simulink library "Energy_converter_Electrical_to_Mechanical"  (R2016a)
settings: Solver=ode1  StartTime=0.0  StopTime=Inf  FixedStep=0.001  RelTol=1e-3
undefined symbols (not defined in the file): API1dcac_efficiency, API2dcac_efficiency, API3dcac_efficiency, aux_power_state, AWR_InvStError, dat, DiscIntNeverNeededParam, EDCU_p_RefTqeMOT, emot_AcCmprFront_inertia, emot_AcCmprFront_nTab_3rdD, emot_AcCmprFront_pwrAC, emot_AcCmprFront_Tau, emot_AcCmprFront_trqTab_2ndD, emot_AcCmprFront_vltTab_1stD, emot_AcCmprRear_inertia, emot_AcCmprRear_nTab_3rdD, emot_AcCmprRear_pwrAC, emot_AcCmprRear_Tau, emot_AcCmprRear_trqTab_2ndD, emot_AcCmprRear_vltTab_1stD, emot_AirCmpr_inertia, emot_AirCmpr_nTab_3rdD, emot_AirCmpr_pwrAC, emot_AirCmpr_Tau, emot_AirCmpr_trqTab_2ndD, emot_AirCmpr_vltTab_1stD, emot_aircomp_power, emot_Cth_rotor, emot_Cth_stator, emot_dtrqEmotNeg, emot_dtrqEmotPtv, emot_inv_pwracTab_1st, emot_inv_pwrDC, emot_inv_pwrLoss, emot_inv_VrmsTab_2nd, emot_j, emot_mot_pwrLoss, emot_nTab_1stD, emot_pwrEtaTab_nRow, emot_pwrEtaTab_pwrTab, emot_pwrEtaTab_trqClm, emot_Rth_rotor_oil, emot_Rth_stator_oil, emot_Rth_stator_rotor, emot_tractiongroup, emot_Trotor_init, emot_trqMaxRow, emot_trqMinRow, emot_Tstator_init, emot_vltTab_3rdD, FirstDrivenAxleNoOfEmot, inv_Cth_cooling_plate, inv_Cth_diode, inv_Cth_IGBT, inv_n_IGBT_per_Switch, inv_Rth_cooling_plate_coolant, inv_Rth_PS_cooling_plate, inv_Tplate_init, inv_Tpowerstack_init, midAxleNoOfEmot ... (+6)
libraries: Electrical_converter x12, Energy_converter_Electrical_to_Mechanical x12, simulink x7
(part 7 of 8)

== system Energy_converter_Electrical_to_Mechanical/AWR_DriveEmot_Gen2/AWR2_3/ZeroWhenNotReady2 ==
  Bus Creator4 : BusCreator  Inputs=11
  zero_EMD3_ACT_DcLinkVoltage : Constant  Value=0
  zero_EMD4_ACT_DcLinkPower : Constant  Value=0
  zero_EMD4_ACT_DigitalInput1 : Constant  Value=0
  zero_EMD4_ACT_InverterState : Constant  Value=0
  zero_EMD4_ACT_MaxJunctionTemperature : Constant  Value=0
  zero_EMD4_ACT_MaximumAvailableTorque : Constant  Value=0
  zero_EMD4_ACT_MotorSpeed : Constant  Value=0
  zero_EMD4_ACT_MotorTemperature : Constant  Value=0
  zero_EMD4_ACT_MotorTorque : Constant  Value=0
  zero_EMD4_ACT_ReferenceTorqueLimited : Constant  Value=0
  zero_trqEmot1DesPhy : Constant  Value=0
  Out1 : Outport
  wires:
  Bus Creator4/1 -> Out1/1  "awr3B"
  zero_EMD3_ACT_DcLinkVoltage/1 -> Bus Creator4/1  "EMD3_ACT_DcLinkVoltage"
  zero_EMD4_ACT_DigitalInput1/1 -> Bus Creator4/2  "EMD_ACT_DigitalInput1"
  zero_EMD4_ACT_MaximumAvailableTorque/1 -> Bus Creator4/3  "EMD_ACT_MaximumAvailableTorque"
  zero_EMD4_ACT_DcLinkPower/1 -> Bus Creator4/4  "EMD_ACT_DcLinkPower"
  zero_EMD4_ACT_MotorSpeed/1 -> Bus Creator4/5  "EMD_ACT_MotorSpeed"
  zero_EMD4_ACT_MotorTorque/1 -> Bus Creator4/6  "EMD_ACT_MotorTorque"
  zero_EMD4_ACT_InverterState/1 -> Bus Creator4/7  "EMD_ACT_InverterState"
  zero_EMD4_ACT_ReferenceTorqueLimited/1 -> Bus Creator4/8  "EMD_ACT_ReferenceTorqueLimited"
  zero_trqEmot1DesPhy/1 -> Bus Creator4/9  "trqEmotDesPhy"
  zero_EMD4_ACT_MaxJunctionTemperature/1 -> Bus Creator4/10  "EMD_ACT_MaxJunctionTemperature"
  zero_EMD4_ACT_MotorTemperature/1 -> Bus Creator4/11  "EMD_ACT_MotorTemperature"

== system Energy_converter_Electrical_to_Mechanical/AWR_DriveEmot_Gen2/EMD1_CMD_Command/Compare To Constant ==
  u : Inport
  Compare : RelationalOperator  Operator===  OutDataTypeStr=boolean  InputSameDT=on
  Constant : Constant  DisableCoverage=on  Value=const  OutDataTypeStr=Inherit: Inherit via back propagation
  y : Outport
  wires:
  Compare/1 -> y/1
  Constant/1 -> Compare/2
  u/1 -> Compare/1

== system Energy_converter_Electrical_to_Mechanical/AWR_DriveEmot_Gen2/EMD1_CMD_Command/Compare To Constant1 ==
  u : Inport
  Compare : RelationalOperator  Operator===  OutDataTypeStr=boolean  InputSameDT=on
  Constant : Constant  DisableCoverage=on  Value=const  OutDataTypeStr=Inherit: Inherit via back propagation
  y : Outport
  wires:
  Compare/1 -> y/1
  Constant/1 -> Compare/2
  u/1 -> Compare/1

== system Energy_converter_Electrical_to_Mechanical/AWR_DriveEmot_Gen2/EMD1_CMD_Command1/Compare To Constant ==
  u : Inport
  Compare : RelationalOperator  Operator===  OutDataTypeStr=boolean  InputSameDT=on
  Constant : Constant  DisableCoverage=on  Value=const  OutDataTypeStr=Inherit: Inherit via back propagation
  y : Outport
  wires:
  Compare/1 -> y/1
  Constant/1 -> Compare/2
  u/1 -> Compare/1

== system Energy_converter_Electrical_to_Mechanical/AWR_DriveEmot_Gen2/EMD1_CMD_Command1/Compare To Constant1 ==
  u : Inport
  Compare : RelationalOperator  Operator===  OutDataTypeStr=boolean  InputSameDT=on
  Constant : Constant  DisableCoverage=on  Value=const  OutDataTypeStr=Inherit: Inherit via back propagation
  y : Outport
  wires:
  Compare/1 -> y/1
  Constant/1 -> Compare/2
  u/1 -> Compare/1

== system Energy_converter_Electrical_to_Mechanical/AWR_DriveEmot_Gen2/EMD1_CMD_Command2/Compare To Constant ==
  u : Inport
  Compare : RelationalOperator  Operator===  OutDataTypeStr=boolean  InputSameDT=on
  Constant : Constant  DisableCoverage=on  Value=const  OutDataTypeStr=Inherit: Inherit via back propagation
  y : Outport
  wires:
  Compare/1 -> y/1
  Constant/1 -> Compare/2
  u/1 -> Compare/1

== system Energy_converter_Electrical_to_Mechanical/AWR_DriveEmot_Gen2/EMD1_CMD_Command2/Compare To Constant1 ==
  u : Inport
  Compare : RelationalOperator  Operator===  OutDataTypeStr=boolean  InputSameDT=on
  Constant : Constant  DisableCoverage=on  Value=const  OutDataTypeStr=Inherit: Inherit via back propagation
  y : Outport
  wires:
  Compare/1 -> y/1
  Constant/1 -> Compare/2
  u/1 -> Compare/1

== system Energy_converter_Electrical_to_Mechanical/AWR_DriveEmot_Gen2/EMD1_CMD_Command3/Compare To Constant ==
  u : Inport
  Compare : RelationalOperator  Operator===  OutDataTypeStr=boolean  InputSameDT=on
  Constant : Constant  DisableCoverage=on  Value=const  OutDataTypeStr=Inherit: Inherit via back propagation
  y : Outport
  wires:
  Compare/1 -> y/1
  Constant/1 -> Compare/2
  u/1 -> Compare/1

== system Energy_converter_Electrical_to_Mechanical/AWR_DriveEmot_Gen2/EMD1_CMD_Command3/Compare To Constant1 ==
  u : Inport
  Compare : RelationalOperator  Operator===  OutDataTypeStr=boolean  InputSameDT=on
  Constant : Constant  DisableCoverage=on  Value=const  OutDataTypeStr=Inherit: Inherit via back propagation
  y : Outport
  wires:
  Compare/1 -> y/1
  Constant/1 -> Compare/2
  u/1 -> Compare/1

== system Energy_converter_Electrical_to_Mechanical/AWR_DriveEmot_Gen2/SummarizeEmotorValuesForVehicle/Avoid_Div_by_zero ==
  U : Inport
  Constant : Constant  Value=10^-6
  Math Function : Math  Operator=reciprocal  SaturateOnIntegerOverflow=on
  Switch : Switch  Criteria=u2 > Threshold
  1/U : Outport
  wires:
  U/1 -> Math Function/1, Switch/2
  Constant/1 -> Switch/3
  Math Function/1 -> Switch/1
  Switch/1 -> 1/U/1

== system Energy_converter_Electrical_to_Mechanical/AWR_DriveEmot_edb_Data/AWR 1 TX/Nm_to_percent ==
  Nm_Torque : Inport
  Reference_Torque : Inport  Port=2
  Constant : Constant  Value=100
  Divide1 : Product  Inputs=*/
  Product1 : Product  RndMeth=Zero
  Torque_Percentage : Outport
  wires:
  Nm_Torque/1 -> Divide1/1  "Nm_Torque"
  Product1/1 -> Torque_Percentage/1  "Torque_Percentage"
  Reference_Torque/1 -> Divide1/2  "Reference_Torque"
  Divide1/1 -> Product1/1
  Constant/1 -> Product1/2

== system Energy_converter_Electrical_to_Mechanical/AWR_DriveEmot_edb_Data/AWR 1 TX/Nm_to_percent1 ==
  Nm_Torque : Inport
  Reference_Torque : Inport  Port=2
  Constant : Constant  Value=100
  Divide1 : Product  Inputs=*/
  Product1 : Product  RndMeth=Zero
  Torque_Percentage : Outport
  wires:
  Constant/1 -> Product1/2
  Divide1/1 -> Product1/1
  Reference_Torque/1 -> Divide1/2  "Reference_Torque"
  Product1/1 -> Torque_Percentage/1  "Torque_Percentage"
  Nm_Torque/1 -> Divide1/1  "Nm_Torque"

== system Energy_converter_Electrical_to_Mechanical/AWR_DriveEmot_edb_Data/AWR 1 TX/Nm_to_percent2 ==
  Nm_Torque : Inport
  Reference_Torque : Inport  Port=2
  Constant : Constant  Value=100
  Divide1 : Product  Inputs=*/
  Product1 : Product  RndMeth=Zero
  Torque_Percentage : Outport
  wires:
  Nm_Torque/1 -> Divide1/1  "Nm_Torque"
  Product1/1 -> Torque_Percentage/1  "Torque_Percentage"
  Reference_Torque/1 -> Divide1/2  "Reference_Torque"
  Divide1/1 -> Product1/1
  Constant/1 -> Product1/2

== system Energy_converter_Electrical_to_Mechanical/AWR_DriveEmot_edb_Data/AWR 2 TX/Nm_to_percent ==
  Nm_Torque : Inport
  Reference_Torque : Inport  Port=2
  Constant : Constant  Value=100
  Divide1 : Product  Inputs=*/
  Product1 : Product  RndMeth=Zero
  Torque_Percentage : Outport
  wires:
  Nm_Torque/1 -> Divide1/1  "Nm_Torque"
  Product1/1 -> Torque_Percentage/1  "Torque_Percentage"
  Reference_Torque/1 -> Divide1/2  "Reference_Torque"
  Divide1/1 -> Product1/1
  Constant/1 -> Product1/2

== system Energy_converter_Electrical_to_Mechanical/AWR_DriveEmot_edb_Data/AWR 2 TX/Nm_to_percent1 ==
  Nm_Torque : Inport
  Reference_Torque : Inport  Port=2
  Constant : Constant  Value=100
  Divide1 : Product  Inputs=*/
  Product1 : Product  RndMeth=Zero
  Torque_Percentage : Outport
  wires:
  Constant/1 -> Product1/2
  Divide1/1 -> Product1/1
  Reference_Torque/1 -> Divide1/2  "Reference_Torque"
  Product1/1 -> Torque_Percentage/1  "Torque_Percentage"
  Nm_Torque/1 -> Divide1/1  "Nm_Torque"

== system Energy_converter_Electrical_to_Mechanical/AWR_DriveEmot_edb_Data/AWR 2 TX/Nm_to_percent2 ==
  Nm_Torque : Inport
  Reference_Torque : Inport  Port=2
  Constant : Constant  Value=100
  Divide1 : Product  Inputs=*/
  Product1 : Product  RndMeth=Zero
  Torque_Percentage : Outport
  wires:
  Nm_Torque/1 -> Divide1/1  "Nm_Torque"
  Product1/1 -> Torque_Percentage/1  "Torque_Percentage"
  Reference_Torque/1 -> Divide1/2  "Reference_Torque"
  Divide1/1 -> Product1/1
  Constant/1 -> Product1/2

== system Energy_converter_Electrical_to_Mechanical/AWR_DriveEmot_edb_Data/AWR 3 TX/Nm_to_percent ==
  Nm_Torque : Inport
  Reference_Torque : Inport  Port=2
  Constant : Constant  Value=100
  Divide1 : Product  Inputs=*/
  Product1 : Product  RndMeth=Zero
  Torque_Percentage : Outport
  wires:
  Constant/1 -> Product1/2
  Divide1/1 -> Product1/1
  Reference_Torque/1 -> Divide1/2  "Reference_Torque"
  Product1/1 -> Torque_Percentage/1  "Torque_Percentage"
  Nm_Torque/1 -> Divide1/1  "Nm_Torque"

== system Energy_converter_Electrical_to_Mechanical/AWR_DriveEmot_edb_Data/AWR 3 TX/Nm_to_percent1 ==
  Nm_Torque : Inport
  Reference_Torque : Inport  Port=2
  Constant : Constant  Value=100
  Divide1 : Product  Inputs=*/
  Product1 : Product  RndMeth=Zero
  Torque_Percentage : Outport
  wires:
  Nm_Torque/1 -> Divide1/1  "Nm_Torque"
  Product1/1 -> Torque_Percentage/1  "Torque_Percentage"
  Reference_Torque/1 -> Divide1/2  "Reference_Torque"
  Divide1/1 -> Product1/1
  Constant/1 -> Product1/2

== system Energy_converter_Electrical_to_Mechanical/AWR_DriveEmot_edb_Data/AWR 3 TX/Nm_to_percent2 ==
  Nm_Torque : Inport
  Reference_Torque : Inport  Port=2
  Constant : Constant  Value=100
  Divide1 : Product  Inputs=*/
  Product1 : Product  RndMeth=Zero
  Torque_Percentage : Outport
  wires:
  Constant/1 -> Product1/2
  Divide1/1 -> Product1/1
  Reference_Torque/1 -> Divide1/2  "Reference_Torque"
  Product1/1 -> Torque_Percentage/1  "Torque_Percentage"
  Nm_Torque/1 -> Divide1/1  "Nm_Torque"

== system Energy_converter_Electrical_to_Mechanical/AWR_DriveEmot_edb_Data/AWR 4 TX/Nm_to_percent ==
  Nm_Torque : Inport
  Reference_Torque : Inport  Port=2
  Constant : Constant  Value=100
  Divide1 : Product  Inputs=*/
  Product1 : Product  RndMeth=Zero
  Torque_Percentage : Outport
  wires:
  Nm_Torque/1 -> Divide1/1  "Nm_Torque"
  Product1/1 -> Torque_Percentage/1  "Torque_Percentage"
  Reference_Torque/1 -> Divide1/2  "Reference_Torque"
  Divide1/1 -> Product1/1
  Constant/1 -> Product1/2

== system Energy_converter_Electrical_to_Mechanical/AWR_DriveEmot_edb_Data/AWR 4 TX/Nm_to_percent1 ==
  Nm_Torque : Inport
  Reference_Torque : Inport  Port=2
  Constant : Constant  Value=100
  Divide1 : Product  Inputs=*/
  Product1 : Product  RndMeth=Zero
  Torque_Percentage : Outport
  wires:
  Constant/1 -> Product1/2
  Divide1/1 -> Product1/1
  Reference_Torque/1 -> Divide1/2  "Reference_Torque"
  Product1/1 -> Torque_Percentage/1  "Torque_Percentage"
  Nm_Torque/1 -> Divide1/1  "Nm_Torque"

== system Energy_converter_Electrical_to_Mechanical/AWR_DriveEmot_edb_Data/AWR 4 TX/Nm_to_percent2 ==
  Nm_Torque : Inport
  Reference_Torque : Inport  Port=2
  Constant : Constant  Value=100
  Divide1 : Product  Inputs=*/
  Product1 : Product  RndMeth=Zero
  Torque_Percentage : Outport
  wires:
  Nm_Torque/1 -> Divide1/1  "Nm_Torque"
  Product1/1 -> Torque_Percentage/1  "Torque_Percentage"
  Reference_Torque/1 -> Divide1/2  "Reference_Torque"
  Divide1/1 -> Product1/1
  Constant/1 -> Product1/2

== system Energy_converter_Electrical_to_Mechanical/AWR_DriveEmot_edb_Data/AWR1_4/ZeroWhenNotReady1 ==
  Bus Creator4 : BusCreator  Inputs=11
  zero_EMD1_ACT_DcLinkPower : Constant  Value=0
  zero_EMD1_ACT_DcLinkVoltage : Constant  Value=0
  zero_EMD1_ACT_DigitalInput1 : Constant  Value=0
  zero_EMD1_ACT_InverterState : Constant  Value=0
  zero_EMD1_ACT_MaxJunctionTemperature : Constant  Value=0
  zero_EMD1_ACT_MaximumAvailableTorque : Constant  Value=0
  zero_EMD1_ACT_MotorSpeed : Constant  Value=0
  zero_EMD1_ACT_MotorTemperature : Constant  Value=0
  zero_EMD1_ACT_MotorTorque : Constant  Value=0
  zero_EMD1_ACT_ReferenceTorqueLimited : Constant  Value=0
  zero_trqEmot1DesPhy : Constant  Value=0
  Out1 : Outport
  wires:
  Bus Creator4/1 -> Out1/1  "awr1B"
  zero_EMD1_ACT_DcLinkVoltage/1 -> Bus Creator4/1  "EMD1_ACT_DcLinkVoltage"
  zero_EMD1_ACT_DigitalInput1/1 -> Bus Creator4/2  "EMD_ACT_DigitalInput1"
  zero_EMD1_ACT_MaximumAvailableTorque/1 -> Bus Creator4/3  "EMD_ACT_MaximumAvailableTorque"
  zero_EMD1_ACT_DcLinkPower/1 -> Bus Creator4/4  "EMD_ACT_DcLinkPower"
  zero_EMD1_ACT_MotorSpeed/1 -> Bus Creator4/5  "EMD_ACT_MotorSpeed"
  zero_EMD1_ACT_MotorTorque/1 -> Bus Creator4/6  "EMD_ACT_MotorTorque"
  zero_EMD1_ACT_InverterState/1 -> Bus Creator4/7  "EMD_ACT_InverterState"
  zero_EMD1_ACT_ReferenceTorqueLimited/1 -> Bus Creator4/8  "EMD_ACT_ReferenceTorqueLimited"
  zero_trqEmot1DesPhy/1 -> Bus Creator4/9  "trqEmotDesPhy"
  zero_EMD1_ACT_MaxJunctionTemperature/1 -> Bus Creator4/10  "EMD_ACT_MaxJunctionTemperature"
  zero_EMD1_ACT_MotorTemperature/1 -> Bus Creator4/11  "EMD_ACT_MotorTemperature"

== system Energy_converter_Electrical_to_Mechanical/AWR_DriveEmot_edb_Data/AWR1_4/ZeroWhenNotReady2 ==
  Bus Creator4 : BusCreator  Inputs=11
  zero_EMD4_ACT_DcLinkPower : Constant  Value=0
  zero_EMD4_ACT_DcLinkVoltage : Constant  Value=0
  zero_EMD4_ACT_DigitalInput1 : Constant  Value=0
  zero_EMD4_ACT_InverterState : Constant  Value=0
  zero_EMD4_ACT_MaxJunctionTemperature : Constant  Value=0
  zero_EMD4_ACT_MaximumAvailableTorque : Constant  Value=0
  zero_EMD4_ACT_MotorSpeed : Constant  Value=0
  zero_EMD4_ACT_MotorTemperature : Constant  Value=0
  zero_EMD4_ACT_MotorTorque : Constant  Value=0
  zero_EMD4_ACT_ReferenceTorqueLimited : Constant  Value=0
  zero_trqEmot1DesPhy : Constant  Value=0
  Out1 : Outport
  wires:
  zero_EMD4_ACT_MotorTemperature/1 -> Bus Creator4/11  "EMD_ACT_MotorTemperature"
  zero_EMD4_ACT_MaxJunctionTemperature/1 -> Bus Creator4/10  "EMD_ACT_MaxJunctionTemperature"
  zero_trqEmot1DesPhy/1 -> Bus Creator4/9  "trqEmotDesPhy"
  zero_EMD4_ACT_ReferenceTorqueLimited/1 -> Bus Creator4/8  "EMD_ACT_ReferenceTorqueLimited"
  zero_EMD4_ACT_InverterState/1 -> Bus Creator4/7  "EMD_ACT_InverterState"
  zero_EMD4_ACT_MotorTorque/1 -> Bus Creator4/6  "EMD_ACT_MotorTorque"
  zero_EMD4_ACT_MotorSpeed/1 -> Bus Creator4/5  "EMD_ACT_MotorSpeed"
  zero_EMD4_ACT_DcLinkPower/1 -> Bus Creator4/4  "EMD_ACT_DcLinkPower"
  zero_EMD4_ACT_MaximumAvailableTorque/1 -> Bus Creator4/3  "EMD_ACT_MaximumAvailableTorque"
  zero_EMD4_ACT_DigitalInput1/1 -> Bus Creator4/2  "EMD_ACT_DigitalInput1"
  zero_EMD4_ACT_DcLinkVoltage/1 -> Bus Creator4/1  "EMD4_ACT_DcLinkVoltage"
  Bus Creator4/1 -> Out1/1  "awr1B"

== system Energy_converter_Electrical_to_Mechanical/AWR_DriveEmot_edb_Data/AWR2_3/ZeroWhenNotReady1 ==
  Bus Creator4 : BusCreator  Inputs=11
  zero_EMD1_ACT_DcLinkPower : Constant  Value=0
  zero_EMD1_ACT_DigitalInput1 : Constant  Value=0
  zero_EMD1_ACT_InverterState : Constant  Value=0
  zero_EMD1_ACT_MaxJunctionTemperature : Constant  Value=0
  zero_EMD1_ACT_MaximumAvailableTorque : Constant  Value=0
  zero_EMD1_ACT_MotorSpeed : Constant  Value=0
  zero_EMD1_ACT_MotorTemperature : Constant  Value=0
  zero_EMD1_ACT_MotorTorque : Constant  Value=0
  zero_EMD1_ACT_ReferenceTorqueLimited : Constant  Value=0
  zero_EMD2_ACT_DcLinkVoltage : Constant  Value=0
  zero_trqEmot1DesPhy : Constant  Value=0
  Out1 : Outport
  wires:
  zero_EMD1_ACT_MotorTemperature/1 -> Bus Creator4/11  "EMD_ACT_MotorTemperature"
  zero_EMD1_ACT_MaxJunctionTemperature/1 -> Bus Creator4/10  "EMD_ACT_MaxJunctionTemperature"
  zero_trqEmot1DesPhy/1 -> Bus Creator4/9  "trqEmotDesPhy"
  zero_EMD1_ACT_ReferenceTorqueLimited/1 -> Bus Creator4/8  "EMD_ACT_ReferenceTorqueLimited"
  zero_EMD1_ACT_InverterState/1 -> Bus Creator4/7  "EMD_ACT_InverterState"
  zero_EMD1_ACT_MotorTorque/1 -> Bus Creator4/6  "EMD_ACT_MotorTorque"
  zero_EMD1_ACT_MotorSpeed/1 -> Bus Creator4/5  "EMD_ACT_MotorSpeed"
  zero_EMD1_ACT_DcLinkPower/1 -> Bus Creator4/4  "EMD_ACT_DcLinkPower"
  zero_EMD1_ACT_MaximumAvailableTorque/1 -> Bus Creator4/3  "EMD_ACT_MaximumAvailableTorque"
  zero_EMD1_ACT_DigitalInput1/1 -> Bus Creator4/2  "EMD_ACT_DigitalInput1"
  zero_EMD2_ACT_DcLinkVoltage/1 -> Bus Creator4/1  "EMD2_ACT_DcLinkVoltage"
  Bus Creator4/1 -> Out1/1  "awr2B"

== system Energy_converter_Electrical_to_Mechanical/AWR_DriveEmot_edb_Data/AWR2_3/ZeroWhenNotReady2 ==
  Bus Creator4 : BusCreator  Inputs=11
  zero_EMD3_ACT_DcLinkVoltage : Constant  Value=0
  zero_EMD4_ACT_DcLinkPower : Constant  Value=0
  zero_EMD4_ACT_DigitalInput1 : Constant  Value=0
  zero_EMD4_ACT_InverterState : Constant  Value=0
  zero_EMD4_ACT_MaxJunctionTemperature : Constant  Value=0
  zero_EMD4_ACT_MaximumAvailableTorque : Constant  Value=0
  zero_EMD4_ACT_MotorSpeed : Constant  Value=0
  zero_EMD4_ACT_MotorTemperature : Constant  Value=0
  zero_EMD4_ACT_MotorTorque : Constant  Value=0
  zero_EMD4_ACT_ReferenceTorqueLimited : Constant  Value=0
  zero_trqEmot1DesPhy : Constant  Value=0
  Out1 : Outport
  wires:
  Bus Creator4/1 -> Out1/1  "awr3B"
  zero_EMD3_ACT_DcLinkVoltage/1 -> Bus Creator4/1  "EMD3_ACT_DcLinkVoltage"
  zero_EMD4_ACT_DigitalInput1/1 -> Bus Creator4/2  "EMD_ACT_DigitalInput1"
  zero_EMD4_ACT_MaximumAvailableTorque/1 -> Bus Creator4/3  "EMD_ACT_MaximumAvailableTorque"
  zero_EMD4_ACT_DcLinkPower/1 -> Bus Creator4/4  "EMD_ACT_DcLinkPower"
  zero_EMD4_ACT_MotorSpeed/1 -> Bus Creator4/5  "EMD_ACT_MotorSpeed"
  zero_EMD4_ACT_MotorTorque/1 -> Bus Creator4/6  "EMD_ACT_MotorTorque"
  zero_EMD4_ACT_InverterState/1 -> Bus Creator4/7  "EMD_ACT_InverterState"
  zero_EMD4_ACT_ReferenceTorqueLimited/1 -> Bus Creator4/8  "EMD_ACT_ReferenceTorqueLimited"
  zero_trqEmot1DesPhy/1 -> Bus Creator4/9  "trqEmotDesPhy"
  zero_EMD4_ACT_MaxJunctionTemperature/1 -> Bus Creator4/10  "EMD_ACT_MaxJunctionTemperature"
  zero_EMD4_ACT_MotorTemperature/1 -> Bus Creator4/11  "EMD_ACT_MotorTemperature"

== system Energy_converter_Electrical_to_Mechanical/AWR_DriveEmot_edb_Data/EMD1_CMD_Command/Compare To Constant ==
  u : Inport
  Compare : RelationalOperator  Operator===  OutDataTypeStr=boolean  InputSameDT=on
  Constant : Constant  DisableCoverage=on  Value=const  OutDataTypeStr=Inherit: Inherit via back propagation
  y : Outport
  wires:
  Compare/1 -> y/1
  Constant/1 -> Compare/2
  u/1 -> Compare/1

== system Energy_converter_Electrical_to_Mechanical/AWR_DriveEmot_edb_Data/EMD1_CMD_Command/Compare To Constant1 ==
  u : Inport
  Compare : RelationalOperator  Operator===  OutDataTypeStr=boolean  InputSameDT=on
  Constant : Constant  DisableCoverage=on  Value=const  OutDataTypeStr=Inherit: Inherit via back propagation
  y : Outport
  wires:
  Compare/1 -> y/1
  Constant/1 -> Compare/2
  u/1 -> Compare/1

== system Energy_converter_Electrical_to_Mechanical/AWR_DriveEmot_edb_Data/EMD1_CMD_Command1/Compare To Constant ==
  u : Inport
  Compare : RelationalOperator  Operator===  OutDataTypeStr=boolean  InputSameDT=on
  Constant : Constant  DisableCoverage=on  Value=const  OutDataTypeStr=Inherit: Inherit via back propagation
  y : Outport
  wires:
  Compare/1 -> y/1
  Constant/1 -> Compare/2
  u/1 -> Compare/1

== system Energy_converter_Electrical_to_Mechanical/AWR_DriveEmot_edb_Data/EMD1_CMD_Command1/Compare To Constant1 ==
  u : Inport
  Compare : RelationalOperator  Operator===  OutDataTypeStr=boolean  InputSameDT=on
  Constant : Constant  DisableCoverage=on  Value=const  OutDataTypeStr=Inherit: Inherit via back propagation
  y : Outport
  wires:
  Compare/1 -> y/1
  Constant/1 -> Compare/2
  u/1 -> Compare/1

== system Energy_converter_Electrical_to_Mechanical/AWR_DriveEmot_edb_Data/EMD1_CMD_Command2/Compare To Constant ==
  u : Inport
  Compare : RelationalOperator  Operator===  OutDataTypeStr=boolean  InputSameDT=on
  Constant : Constant  DisableCoverage=on  Value=const  OutDataTypeStr=Inherit: Inherit via back propagation
  y : Outport
  wires:
  Compare/1 -> y/1
  Constant/1 -> Compare/2
  u/1 -> Compare/1

== system Energy_converter_Electrical_to_Mechanical/AWR_DriveEmot_edb_Data/EMD1_CMD_Command2/Compare To Constant1 ==
  u : Inport
  Compare : RelationalOperator  Operator===  OutDataTypeStr=boolean  InputSameDT=on
  Constant : Constant  DisableCoverage=on  Value=const  OutDataTypeStr=Inherit: Inherit via back propagation
  y : Outport
  wires:
  Compare/1 -> y/1
  Constant/1 -> Compare/2
  u/1 -> Compare/1

== system Energy_converter_Electrical_to_Mechanical/AWR_DriveEmot_edb_Data/EMD1_CMD_Command3/Compare To Constant ==
  u : Inport
  Compare : RelationalOperator  Operator===  OutDataTypeStr=boolean  InputSameDT=on
  Constant : Constant  DisableCoverage=on  Value=const  OutDataTypeStr=Inherit: Inherit via back propagation
  y : Outport
  wires:
  Compare/1 -> y/1
  Constant/1 -> Compare/2
  u/1 -> Compare/1

== system Energy_converter_Electrical_to_Mechanical/AWR_DriveEmot_edb_Data/EMD1_CMD_Command3/Compare To Constant1 ==
  u : Inport
  Compare : RelationalOperator  Operator===  OutDataTypeStr=boolean  InputSameDT=on
  Constant : Constant  DisableCoverage=on  Value=const  OutDataTypeStr=Inherit: Inherit via back propagation
  y : Outport
  wires:
  Compare/1 -> y/1
  Constant/1 -> Compare/2
  u/1 -> Compare/1

== system Energy_converter_Electrical_to_Mechanical/AWR_DriveEmot_edb_Data/SummarizeEmotorValuesForVehicle/Avoid_Div_by_zero ==
  U : Inport
  Constant : Constant  Value=10^-6
  Math Function : Math  Operator=reciprocal  SaturateOnIntegerOverflow=on
  Switch : Switch  Criteria=u2 > Threshold
  1/U : Outport
  wires:
  U/1 -> Math Function/1, Switch/2
  Constant/1 -> Switch/3
  Math Function/1 -> Switch/1
  Switch/1 -> 1/U/1

== system Energy_converter_Electrical_to_Mechanical/GTR_Electric_machine/Thermal/Cooling2 ==
  power loss : Inport
  cooling inlet : Inport  Port=2
  Add1 : Sum  Inputs=-+
  Add2 : Sum  Inputs=-+
  Bus Selector : BusSelector  OutputSignals=mass flow [kg/s],temperature [K]
  Gain : Gain  Gain=1/dat.Rth.value
  Gain1 : Gain  Gain=1/dat.cm.value
  Integrator : Integrator  InitialCondition=hilsmdl.init.temp.value
  Mux : Mux  Inputs=3
  Mux1 : Mux  Inputs=2
  calc mean temperature : Fcn  Expr=dat.alpha.value*u(1) + (1-dat.alpha.value)*u(2)
  calc outlet temperature : Fcn  Expr=(u(3)+u(2)*(dat.Rth.value*dat.coolingFluid.c.value*u(1)-dat.alpha.value)) / (1+dat.Rth.value*dat.coolingFluid.c.value*u(1)-dat.alpha.value)
  internal temperature : Outport
  fluid outlet temperature : Outport  Port=2
  wires:
  Mux/1 -> calc outlet temperature/1
  calc outlet temperature/1 -> Mux1/2, fluid outlet temperature/1  "fluid outlet temperature [K]"
  Bus Selector/2 -> Mux1/1, Mux/2  "<temperature [K]>"
  Add1/1 -> Gain/1
  Gain/1 -> Add2/1  "P cooling [W]"
  Add2/1 -> Gain1/1
  Gain1/1 -> Integrator/1
  Integrator/1 -> Mux/3, Add1/2, internal temperature/1  "internal temperature [K]"
  cooling inlet/1 -> Bus Selector/1
  power loss/1 -> Add2/2  "power loss [W]"
  Mux1/1 -> calc mean temperature/1
  calc mean temperature/1 -> Add1/1  "T_mean [K]"
  Bus Selector/1 -> Mux/1  "<mass flow [kg/s]>"

== system Energy_converter_Electrical_to_Mechanical/GTR_Electric_machine/local controller/PI controller ==
  RefSpeed : Inport
  ActSpeed : Inport  Port=2
  Reset : Inport  Port=3
  Gain : Gain  Gain=dat.controller.i.value
  Gain2 : Gain  Gain=dat.controller.p.value
  Integrator : Integrator  ExternalReset=either
  Product : Product  RndMeth=Zero
  Sum : Sum  Inputs=|+-
  Sum1 : Sum  Inputs=|++
  Ctrl signal : Outport
  wires:
  Sum1/1 -> Ctrl signal/1
  Reset/1 -> Integrator/2, Product/2
  ActSpeed/1 -> Sum/2
  RefSpeed/1 -> Sum/1
  Product/1 -> Integrator/1
  Gain/1 -> Product/1
  Gain2/1 -> Sum1/2
  Integrator/1 -> Sum1/1
  Sum/1 -> Gain2/1, Gain/1

== system Energy_converter_Electrical_to_Mechanical/e-Motor/Thermic_Model_Inverter/C_IGBT_and_Diode ==
  P_Heat_eff : Inport
  T : Inport  Port=2
  Add : Sum
  Clock : Clock
  Divide : Product  Inputs=*/
  Heat_Capacity_PowerStack [J/K] : Constant  Value=inv_Cth_IGBT+inv_Cth_diode
  Product : Product
  Product1 : Product
  Sum : Sum  Inputs=|+-
  Unit Delay : UnitDelay  SampleTime=-1
  T_new : Outport
  wires:
  Sum/1 -> Product/2  "[s]"
  P_Heat_eff/1 -> Product/1
  Product/1 -> Add/1  "[J]"
  T/1 -> Product1/1  "[K]"
  Heat_Capacity_PowerStack [J/K]/1 -> Product1/2, Divide/2
  Product1/1 -> Add/2  "[J]"
  Add/1 -> Divide/1
  Divide/1 -> T_new/1  "[K]"
  Clock/1 -> Sum/1, Unit Delay/1
  Unit Delay/1 -> Sum/2

== system Energy_converter_Electrical_to_Mechanical/e-Motor/Thermic_Model_Inverter/C_Plate ==
  P_Heat_eff : Inport
  T : Inport  Port=2
  Add : Sum
  Clock : Clock
  Divide : Product  Inputs=*/
  Heat_Capacity_Plate [J/K] : Constant  Value=inv_Cth_cooling_plate
  Product : Product
  Product1 : Product
  Sum : Sum  Inputs=|+-
  Unit Delay : UnitDelay  SampleTime=-1
  T_new : Outport
  wires:
  Sum/1 -> Product/2  "[s]"
  P_Heat_eff/1 -> Product/1
  Product/1 -> Add/1  "[J]"
  T/1 -> Product1/1  "[K]"
  Product1/1 -> Add/2  "[J]"
  Add/1 -> Divide/1
  Divide/1 -> T_new/1  "[K]"
  Heat_Capacity_Plate [J/K]/1 -> Product1/2, Divide/2
  Clock/1 -> Sum/1, Unit Delay/1
  Unit Delay/1 -> Sum/2

== system Energy_converter_Electrical_to_Mechanical/e-Motor/Thermic_Model_Inverter/R_PS-Plate ==
  T_IGBT : Inport
  T_Plate : Inport  Port=2
  Add : Sum  Inputs=+-
  Divide : Product  Inputs=*/
  R_th_IGBT_Plate : Constant  Value=inv_Rth_PS_cooling_plate
  dQ : Outport
  wires:
  R_th_IGBT_Plate/1 -> Divide/2
  Divide/1 -> dQ/1
  Add/1 -> Divide/1
  T_Plate/1 -> Add/2
  T_IGBT/1 -> Add/1

== system Energy_converter_Electrical_to_Mechanical/e-Motor/Thermic_Model_Inverter/R_Plate-Coolant ==
  T_Plate : Inport
  T_Coolant : Inport  Port=2
  Add : Sum  Inputs=+-
  Divide : Product  Inputs=*/
  Rth_cooling_plate_coolant : Constant  Value=inv_Rth_cooling_plate_coolant
  dQ : Outport
  wires:
  T_Plate/1 -> Add/1
  T_Coolant/1 -> Add/2
  Add/1 -> Divide/1
  Divide/1 -> dQ/1
  Rth_cooling_plate_coolant/1 -> Divide/2

== system Energy_converter_Electrical_to_Mechanical/e-Motor/Thermic_Model_PMSM_slot2/C_Rotor ==
  P_Heat_eff : Inport
  T : Inport  Port=2
  Add : Sum
  Clock : Clock
  Divide : Product  Inputs=*/
  Heat_Capacity_Rotor [J/K] : Constant  Value=emot_Cth_rotor
  Product : Product
  Product1 : Product
  Sum : Sum  Inputs=|+-
  Unit Delay : UnitDelay  SampleTime=-1
  T_new : Outport
  wires:
  Divide/1 -> T_new/1  "[K]"
  Add/1 -> Divide/1
  Product1/1 -> Add/2  "[J]"
  Heat_Capacity_Rotor [J/K]/1 -> Divide/2, Product1/2
  T/1 -> Product1/1  "[K]"
  Product/1 -> Add/1  "[J]"
  P_Heat_eff/1 -> Product/1
  Sum/1 -> Product/2  "[s]"
  Clock/1 -> Sum/1, Unit Delay/1
  Unit Delay/1 -> Sum/2

== system Energy_converter_Electrical_to_Mechanical/e-Motor/Thermic_Model_PMSM_slot2/C_Stator ==
  P_Heat_eff : Inport
  T : Inport  Port=2
  Add : Sum
  Clock : Clock
  Divide : Product  Inputs=*/
  Heat_Capacity_Stator [J/K] : Constant  Value=emot_Cth_stator
  Product : Product
  Product1 : Product
  Sum : Sum  Inputs=|+-
  Unit Delay : UnitDelay  SampleTime=-1
  T_new : Outport
  wires:
  Sum/1 -> Product/2  "[s]"
  P_Heat_eff/1 -> Product/1
  Product/1 -> Add/1  "[J]"
  T/1 -> Product1/1  "[K]"
  Heat_Capacity_Stator [J/K]/1 -> Product1/2, Divide/2
  Product1/1 -> Add/2  "[J]"
  Add/1 -> Divide/1
  Divide/1 -> T_new/1  "[K]"
  Clock/1 -> Sum/1, Unit Delay/1
  Unit Delay/1 -> Sum/2

== system Energy_converter_Electrical_to_Mechanical/e-Motor/Thermic_Model_PMSM_slot2/K2degC ==
  In1 : Inport
  Add : Sum  Inputs=+-
  Constant : Constant  Value=273.15
  Out1 : Outport
  wires:
  In1/1 -> Add/1
  Add/1 -> Out1/1
  Constant/1 -> Add/2

== system Energy_converter_Electrical_to_Mechanical/e-Motor/Thermic_Model_PMSM_slot2/K2degC1 ==
  In1 : Inport
  Add : Sum  Inputs=+-
  Constant : Constant  Value=273.15
  Out1 : Outport
  wires:
  In1/1 -> Add/1
  Add/1 -> Out1/1
  Constant/1 -> Add/2

== system Energy_converter_Electrical_to_Mechanical/e-Motor/Thermic_Model_PMSM_slot2/R_RotorOil ==
  T_Rotor : Inport
  T_Oil : Inport  Port=2
  Add : Sum  Inputs=+-
  Divide : Product  Inputs=*/
  R_th_Rot_Oil : Constant  Value=emot_Rth_rotor_oil
  dQ : Outport
  wires:
  T_Rotor/1 -> Add/1
  T_Oil/1 -> Add/2
  Add/1 -> Divide/1
  Divide/1 -> dQ/1
  R_th_Rot_Oil/1 -> Divide/2

== system Energy_converter_Electrical_to_Mechanical/e-Motor/Thermic_Model_PMSM_slot2/R_StatorOil ==
  T_Oil : Inport
  T_Stator : Inport  Port=2
  Add : Sum  Inputs=-+
  Divide : Product  Inputs=*/
  R_th_Stat_Oil : Constant  Value=emot_Rth_stator_oil
  dQ : Outport
  wires:
  T_Oil/1 -> Add/1
  T_Stator/1 -> Add/2
  Add/1 -> Divide/1
  Divide/1 -> dQ/1
  R_th_Stat_Oil/1 -> Divide/2

== system Energy_converter_Electrical_to_Mechanical/e-Motor/Thermic_Model_PMSM_slot2/R_StatorRotor ==
  T_Stator : Inport
  T_Rotor : Inport  Port=2
  Add : Sum  Inputs=+-
  Divide : Product  Inputs=*/
  R_th_Stat_Rot : Constant  Value=emot_Rth_stator_rotor
  dQ : Outport
  wires:
  R_th_Stat_Rot/1 -> Divide/2
  Divide/1 -> dQ/1
  Add/1 -> Divide/1
  T_Rotor/1 -> Add/2
  T_Stator/1 -> Add/1

== system Energy_converter_Electrical_to_Mechanical/e-Motor/Thermic_Model_PMSM_slot2/degC2K ==
  In1 : Inport
  Add : Sum
  Constant : Constant  Value=273.15
  Out1 : Outport
  wires:
  In1/1 -> Add/1
  Add/1 -> Out1/1
  Constant/1 -> Add/2

== system Energy_converter_Electrical_to_Mechanical/e-Motor/Thermic_Model_PMSM_slot2/degC2K1 ==
  In1 : Inport
  Add : Sum
  Constant : Constant  Value=273.15
  Out1 : Outport
  wires:
  Constant/1 -> Add/2
  Add/1 -> Out1/1
  In1/1 -> Add/1

== system Energy_converter_Electrical_to_Mechanical/e-Motor/Thermic_Model_PMSM_slot2/degC2K2 ==
  In1 : Inport
  Add : Sum
  Constant : Constant  Value=273.15
  Out1 : Outport
  wires:
  In1/1 -> Add/1
  Add/1 -> Out1/1
  Constant/1 -> Add/2

== system Energy_converter_Electrical_to_Mechanical/e-Motor_Gen2/Thermic_Model_Inverter/C_IGBT_and_Diode ==
  P_Heat_eff : Inport
  T : Inport  Port=2
  Add : Sum
  Clock : Clock
  Divide : Product  Inputs=*/
  Heat_Capacity_PowerStack [J/K] : Constant  Value=inv_Cth_IGBT+inv_Cth_diode
  Product : Product
  Product1 : Product
  Sum : Sum  Inputs=|+-
  Unit Delay : UnitDelay  SampleTime=-1
  T_new : Outport
  wires:
  Sum/1 -> Product/2  "[s]"
  P_Heat_eff/1 -> Product/1
  Product/1 -> Add/1  "[J]"
  T/1 -> Product1/1  "[K]"
  Heat_Capacity_PowerStack [J/K]/1 -> Product1/2, Divide/2
  Product1/1 -> Add/2  "[J]"
  Add/1 -> Divide/1
  Divide/1 -> T_new/1  "[K]"
  Clock/1 -> Sum/1, Unit Delay/1
  Unit Delay/1 -> Sum/2

== system Energy_converter_Electrical_to_Mechanical/e-Motor_Gen2/Thermic_Model_Inverter/C_Plate ==
  P_Heat_eff : Inport
  T : Inport  Port=2
  Add : Sum
  Clock : Clock
  Divide : Product  Inputs=*/
  Heat_Capacity_Plate [J/K] : Constant  Value=inv_Cth_cooling_plate
  Product : Product
  Product1 : Product
  Sum : Sum  Inputs=|+-
  Unit Delay : UnitDelay  SampleTime=-1
  T_new : Outport
  wires:
  Sum/1 -> Product/2  "[s]"
  P_Heat_eff/1 -> Product/1
  Product/1 -> Add/1  "[J]"
  T/1 -> Product1/1  "[K]"
  Product1/1 -> Add/2  "[J]"
  Add/1 -> Divide/1
  Divide/1 -> T_new/1  "[K]"
  Heat_Capacity_Plate [J/K]/1 -> Product1/2, Divide/2
  Clock/1 -> Sum/1, Unit Delay/1
  Unit Delay/1 -> Sum/2

== system Energy_converter_Electrical_to_Mechanical/e-Motor_Gen2/Thermic_Model_Inverter/R_PS-Plate ==
  T_IGBT : Inport
  T_Plate : Inport  Port=2
  Add : Sum  Inputs=+-
  Divide : Product  Inputs=*/
  R_th_IGBT_Plate : Constant  Value=inv_Rth_PS_cooling_plate
  dQ : Outport
  wires:
  R_th_IGBT_Plate/1 -> Divide/2
  Divide/1 -> dQ/1
  Add/1 -> Divide/1
  T_Plate/1 -> Add/2
  T_IGBT/1 -> Add/1

== system Energy_converter_Electrical_to_Mechanical/e-Motor_Gen2/Thermic_Model_Inverter/R_Plate-Coolant ==
  T_Plate : Inport
  T_Coolant : Inport  Port=2
  Add : Sum  Inputs=+-
  Divide : Product  Inputs=*/
  Rth_cooling_plate_coolant : Constant  Value=inv_Rth_cooling_plate_coolant
  dQ : Outport
  wires:
  T_Plate/1 -> Add/1
  T_Coolant/1 -> Add/2
  Add/1 -> Divide/1
  Divide/1 -> dQ/1
  Rth_cooling_plate_coolant/1 -> Divide/2

== system Energy_converter_Electrical_to_Mechanical/e-Motor_Gen2/Thermic_Model_PMSM_slot2/C_Rotor ==
  P_Heat_eff : Inport
  T : Inport  Port=2
  Add : Sum
  Clock : Clock
  Divide : Product  Inputs=*/
  Heat_Capacity_Rotor [J/K] : Constant  Value=emot_Cth_rotor
  Product : Product
  Product1 : Product
  Sum : Sum  Inputs=|+-
  Unit Delay : UnitDelay  SampleTime=-1
  T_new : Outport
  wires:
  Divide/1 -> T_new/1  "[K]"
  Add/1 -> Divide/1
  Product1/1 -> Add/2  "[J]"
  Heat_Capacity_Rotor [J/K]/1 -> Divide/2, Product1/2
  T/1 -> Product1/1  "[K]"
  Product/1 -> Add/1  "[J]"
  P_Heat_eff/1 -> Product/1
  Sum/1 -> Product/2  "[s]"
  Clock/1 -> Sum/1, Unit Delay/1
  Unit Delay/1 -> Sum/2

== system Energy_converter_Electrical_to_Mechanical/e-Motor_Gen2/Thermic_Model_PMSM_slot2/C_Stator ==
  P_Heat_eff : Inport
  T : Inport  Port=2
  Add : Sum
  Clock : Clock
  Divide : Product  Inputs=*/
  Heat_Capacity_Stator [J/K] : Constant  Value=emot_Cth_stator
  Product : Product
  Product1 : Product
  Sum : Sum  Inputs=|+-
  Unit Delay : UnitDelay  SampleTime=-1
  T_new : Outport
  wires:
  Sum/1 -> Product/2  "[s]"
  P_Heat_eff/1 -> Product/1
  Product/1 -> Add/1  "[J]"
  T/1 -> Product1/1  "[K]"
  Heat_Capacity_Stator [J/K]/1 -> Product1/2, Divide/2
  Product1/1 -> Add/2  "[J]"
  Add/1 -> Divide/1
  Divide/1 -> T_new/1  "[K]"
  Clock/1 -> Sum/1, Unit Delay/1
  Unit Delay/1 -> Sum/2

== system Energy_converter_Electrical_to_Mechanical/e-Motor_Gen2/Thermic_Model_PMSM_slot2/K2degC ==
  In1 : Inport
  Add : Sum  Inputs=+-
  Constant : Constant  Value=273.15
  Out1 : Outport
  wires:
  In1/1 -> Add/1
  Add/1 -> Out1/1
  Constant/1 -> Add/2

== system Energy_converter_Electrical_to_Mechanical/e-Motor_Gen2/Thermic_Model_PMSM_slot2/K2degC1 ==
  In1 : Inport
  Add : Sum  Inputs=+-
  Constant : Constant  Value=273.15
  Out1 : Outport
  wires:
  In1/1 -> Add/1
  Add/1 -> Out1/1
  Constant/1 -> Add/2

== system Energy_converter_Electrical_to_Mechanical/e-Motor_Gen2/Thermic_Model_PMSM_slot2/R_RotorOil ==
  T_Rotor : Inport
  T_Oil : Inport  Port=2
  Add : Sum  Inputs=+-
  Divide : Product  Inputs=*/
  R_th_Rot_Oil : Constant  Value=emot_Rth_rotor_oil
  dQ : Outport
  wires:
  T_Rotor/1 -> Add/1
  T_Oil/1 -> Add/2
  Add/1 -> Divide/1
  Divide/1 -> dQ/1
  R_th_Rot_Oil/1 -> Divide/2

== system Energy_converter_Electrical_to_Mechanical/e-Motor_Gen2/Thermic_Model_PMSM_slot2/R_StatorOil ==
  T_Oil : Inport
  T_Stator : Inport  Port=2
  Add : Sum  Inputs=-+
  Divide : Product  Inputs=*/
  R_th_Stat_Oil : Constant  Value=emot_Rth_stator_oil
  dQ : Outport
  wires:
  T_Oil/1 -> Add/1
  T_Stator/1 -> Add/2
  Add/1 -> Divide/1
  Divide/1 -> dQ/1
  R_th_Stat_Oil/1 -> Divide/2

== system Energy_converter_Electrical_to_Mechanical/e-Motor_Gen2/Thermic_Model_PMSM_slot2/R_StatorRotor ==
  T_Stator : Inport
  T_Rotor : Inport  Port=2
  Add : Sum  Inputs=+-
  Divide : Product  Inputs=*/
  R_th_Stat_Rot : Constant  Value=emot_Rth_stator_rotor
  dQ : Outport
  wires:
  R_th_Stat_Rot/1 -> Divide/2
  Divide/1 -> dQ/1
  Add/1 -> Divide/1
  T_Rotor/1 -> Add/2
  T_Stator/1 -> Add/1

== system Energy_converter_Electrical_to_Mechanical/e-Motor_Gen2/Thermic_Model_PMSM_slot2/degC2K ==
  In1 : Inport
  Add : Sum
  Constant : Constant  Value=273.15
  Out1 : Outport
  wires:
  In1/1 -> Add/1
  Add/1 -> Out1/1
  Constant/1 -> Add/2

== system Energy_converter_Electrical_to_Mechanical/e-Motor_Gen2/Thermic_Model_PMSM_slot2/degC2K1 ==
  In1 : Inport
  Add : Sum
  Constant : Constant  Value=273.15
  Out1 : Outport
  wires:
  Constant/1 -> Add/2
  Add/1 -> Out1/1
  In1/1 -> Add/1

== system Energy_converter_Electrical_to_Mechanical/e-Motor_Gen2/Thermic_Model_PMSM_slot2/degC2K2 ==
  In1 : Inport
  Add : Sum
  Constant : Constant  Value=273.15
  Out1 : Outport
  wires:
  In1/1 -> Add/1
  Add/1 -> Out1/1
  Constant/1 -> Add/2

== system Energy_converter_Electrical_to_Mechanical/e-Motor_Gen2/Umrichter mit trq-Regler/Voltage_Calc ==
  RPM : Inport
  Trq : Inport  Port=2
  2-D Lookup Table3 : Lookup_n-D  NumberOfTableDimensions=1  BreakpointsForDimension1=emot_nTab_1stD  BreakpointsForDimension2=[1:3]  Table=Trq_Nm_eMotor_Continuous  RndMeth=Simplest  InputSameDT=on
  2-D Lookup Table4 : Lookup_n-D  BreakpointsForDimension1=emot_nTab_1stD  BreakpointsForDimension2=[0:1]  Table=[Voltage_V_eMotor_Peak ; Voltage_V_eMotor_Continuous]'  RndMeth=Simplest  InputSameDT=on
  Abs1 : Abs
  Data Type Conversion : DataTypeConversion
  Relational Operator : RelationalOperator  Operator=<=  OutDataTypeStr=boolean
  V_rms : Outport
  wires:
  Data Type Conversion/1 -> 2-D Lookup Table4/2
  Abs1/1 -> Relational Operator/2
  Relational Operator/1 -> Data Type Conversion/1
  2-D Lookup Table3/1 -> Relational Operator/1
  RPM/1 -> 2-D Lookup Table3/1, 2-D Lookup Table4/1
  Trq/1 -> Abs1/1
  2-D Lookup Table4/1 -> V_rms/1

== system Energy_converter_Electrical_to_Mechanical/e-Motor_chy_proposal/Umrichter mit trq-Regler/Rate Limiter Dynamic ==
  note: Y(k)
  note: U(k)
  up : Inport
  u : Inport  Port=2
  lo : Inport  Port=3
  Delay Input2 : UnitDelay  Description=Store in Global RAM  DisableCoverage=on  SampleTime=-1
  Difference Inputs1 : Sum  Description=Add in CPU  DisableCoverage=on  Inputs=+-  OutDataTypeStr=Inherit: Inherit via back propagation
  Difference Inputs2 : Sum  Description=Add in CPU  OutDataTypeStr=Inherit: Inherit via back propagation
  FixPt Data Type Duplicate : DataTypeDuplicate  DisableCoverage=on  NumInputPorts=7
  Saturation Dynamic : Subsystem  mask(Saturation Dynamic){OutMin=[], OutMax=[], OutDataTypeStr=Inherit: Same as second input, OutputDataTypeScalingMode=Same as second input, OutDataType=fixdt(1, 16), OutScaling=2^-10, LockScale=off, RndMeth=Floor, DoSatur=off}
      mask prompts: OutMin "Simulink:masks:OutputMinimum_MP"; OutMax "Simulink:masks:OutputMaximum_MP"; OutDataTypeStr "Simulink:masks:OutputDataType_MP"; OutputDataTypeScalingMode "Simulink:masks:OutputDataTypeMode_MP"; OutDataType "Simulink:masks:OutputDataTypeegFixdt116Fixdtsingle_MP"; OutScaling "Simulink:masks:OutputScalingSlopeEg29OrSlopeBias_MP"; LockScale "Simulink:masks:LockOutputDataTypeAgainstFxpTools_MP"; RndMeth "Simulink:masks:IntegerRoundingMode_MP"; DoSatur "Simulink:masks:SaturateOnIntegerOverflow_MP"
      mask help: Simulink:masks:SaturationDynamic_MD
      mask init: same as Energy_converter_Electrical_to_Mechanical/e-Motor_chy_proposal/Umrichter mit trq-Regler/Saturation Dynamic
      mask Callback OutDataTypeStr: fixptdialog(gcbh)
      mask TypeOptions OutputDataTypeScalingMode: double | single | int8 | uint8 | int16 | uint16 | int32 | uint32 | Specify via dialog | Same as second input
      mask Callback OutputDataTypeScalingMode: fixptdialog(gcbh)
      mask Callback OutDataType: fixptdialog(gcbh)
      mask TypeOptions RndMeth: Simulink:masks:Ceiling | Simulink:masks:Convergent | Simulink:masks:Floor | Simulink:masks:Nearest | Simulink:masks:Round | Simulink:masks:Simplest | Simulink:masks:Zero
      mask Display: plot([0.15 0.85],[.5 .5],[.5 .5],[0.05 0.95],0.15+0.7*[0 .25 .75 1],0.05+0.9*[.25 .25 .75 .75]);
  delta fall limit : Product  DisableCoverage=on  Inputs=**  OutDataTypeStr=Inherit: Inherit via back propagation  SaturateOnIntegerOverflow=on
  delta rise limit : Product  DisableCoverage=on  Inputs=**  OutDataTypeStr=Inherit: Inherit via back propagation  SaturateOnIntegerOverflow=on
  sample time : SampleTimeMath  DisableCoverage=on  TsampMathOp=Ts Only  weightValue=1
  Y : Outport  InitialOutput=0
  wires:
  Difference Inputs1/1 -> FixPt Data Type Duplicate/4, Saturation Dynamic/2(u)  "( U(k) - Y(k-1) )"
  u/1 -> Difference Inputs1/1, FixPt Data Type Duplicate/5, sample time/1
  delta fall limit/1 -> FixPt Data Type Duplicate/3, Saturation Dynamic/3(lo)
  Saturation Dynamic/1(y) -> Difference Inputs2/1, FixPt Data Type Duplicate/7
  Delay Input2/1 -> Difference Inputs2/2, Difference Inputs1/2, FixPt Data Type Duplicate/2  "Y(k-1)"
  Difference Inputs2/1 -> Y/1, Delay Input2/1, FixPt Data Type Duplicate/1
  up/1 -> delta rise limit/1
  delta rise limit/1 -> FixPt Data Type Duplicate/6, Saturation Dynamic/1(up)
  lo/1 -> delta fall limit/1
  sample time/1 -> delta fall limit/2, delta rise limit/2

== system Energy_converter_Electrical_to_Mechanical/e-Motor_chy_proposal/Umrichter mit trq-Regler/Saturation Dynamic ==
  up : Inport
  u : Inport  Port=2
  lo : Inport  Port=3
  Data Type Duplicate : DataTypeDuplicate  DisableCoverage=on
  Data Type Propagation : S-Function  FunctionName=sfix_dtprop  Parameters=14,PropDataTypeMode,(getdatatypespecs(PropDataType,PropScaling,DblOver,0, 0, PropDataTypeMode, PropScalingMode)),IfRefDouble,IfRefSingle,IsSigned,NumBitsBase,NumBitsMult,NumBitsAdd,(sort(reshape(round(NumBitsAllowFinal), prod(size(NumBitsAllowFinal)),1))),PropScalingMode,ValuesUsedBestPrec,SlopeBase,SlopeMult,SlopeAdd,BiasBase,BiasMult,BiasAdd,DblOver  SFunctionDeploymentMode=off  EnableBusSupport=off  mask(Data Type Propagation){PropDataTypeMode=Inherit via propagation rule, PropDataType=fixdt(1, 16), IfRefDouble=double, IfRefSingle=single, IsSigned=IsSigned1, NumBitsBase=NumBits1, NumBitsMult=1, NumBitsAdd=0, NumBitsAllowFinal=1:128, PropScalingMode=Inherit via propagation rule, PropScaling=2^-10, ValuesUsedBestPrec=[5 -7], SlopeBase=Slope1, SlopeMult=1, SlopeAdd=0, BiasBase=Bias1, BiasMult=1, BiasAdd=0}
      mask prompts: PropDataTypeMode "Simulink:masks:x1PropagatedDataType_MP"; PropDataType "Simulink:masks:x11PropagatedDataTypeegFixdt116Fixdtsingle_MP"; IfRefDouble "Simulink:masks:x11IfAnyReferenceInputIsDoubleOutputIs_MP"; IfRefSingle "Simulink:masks:x12IfAnyReferenceInputIsSingleOutputIs_MP"; IsSigned "Simulink:masks:x13IsSigned_MP"; NumBitsBase "Simulink:masks:x141NumberofBitsBase_MP"; NumBitsMult "Simulink:masks:x142NumberofBitsMultiplicativeAdjustment_MP"; NumBitsAdd "Simulink:masks:x143NumberofBitsAdditiveAdjustment_MP"; NumBitsAllowFinal "Simulink:masks:x144NumberofBitsAllowableFinalValues_MP"; PropScalingMode "Simulink:masks:x2PropagatedScaling_MP"; PropScaling "Simulink:masks:x21PropagatedScalingSlopeEg29OrSlopeBiasEg1253_MP"; ValuesUsedBestPrec "Simulink:masks:x21ValuesUsedToDetermineBestPrecisionScaling_MP"; SlopeBase "Simulink:masks:x211SlopeBase_MP"; SlopeMult "Simulink:masks:x212SlopeMultiplicativeAdjustment_MP"; SlopeAdd "Simulink:masks:x213SlopeAdditiveAdjustment_MP"; BiasBase "Simulink:masks:x221BiasBase_MP"; BiasMult "Simulink:masks:x222BiasMultiplicativeAdjustment_MP"; BiasAdd "Simulink:masks:x223BiasAdditiveAdjustment_MP"
      mask help: Simulink:masks:DataTypePropagation_MD
      mask init:
      | DblOver = 0;
      mask TypeOptions PropDataTypeMode: Simulink:masks:SpecifyViaDialog | Simulink:masks:InheritViaPropagationRule
      mask Callback PropDataTypeMode: fixptdialog(gcbh)
      mask Callback PropDataType: fixptdialog(gcbh)
      mask TypeOptions IfRefDouble: Simulink:masks:double | Simulink:masks:single
      mask TypeOptions IfRefSingle: Simulink:masks:double | Simulink:masks:single
      mask TypeOptions IsSigned: Simulink:masks:IsSigned1 | Simulink:masks:IsSigned2 | Simulink:masks:IsSigned1OrIsSigned2 | Simulink:masks:TRUE | Simulink:masks:FALSE
      mask TypeOptions NumBitsBase: NumBits1 | NumBits2 | max([NumBits1 NumBits2]) | min([NumBits1 NumBits2]) | NumBits1+NumBits2
      mask TypeOptions PropScalingMode: Simulink:masks:SpecifyViaDialog | Simulink:masks:InheritViaPropagationRule | Simulink:masks:ObtainViaBestPrecision
      mask Callback PropScalingMode: fixptdialog(gcbh)
      mask TypeOptions SlopeBase: Slope1 | Slope2 | max([Slope1 Slope2]) | min([Slope1 Slope2]) | Slope1*Slope2 | Slope1/Slope2 | PosRange1 | PosRange2 | max([PosRange1 PosRange2]) | min([PosRange1 PosRange2]) | PosRange1*PosRange2 | PosRange1/PosRange2
      mask TypeOptions BiasBase: Bias1 | Bias2 | max([Bias1 Bias2]) | min([Bias1 Bias2]) | Bias1*Bias2 | Bias1/Bias2 | Bias1+Bias2 | Bias1-Bias2
      mask Display:
      | port_label('Input',1,'Ref1');
      | port_label('Input',2,'Ref2');
      | port_label('Input',3,'Prop');
  LowerRelop1 : RelationalOperator  DisableCoverage=on  Operator=>  OutDataTypeStr=boolean
  Switch : Switch  Criteria=u2 ~= 0  OutDataTypeStr=Inherit: Inherit via back propagation  ZeroCross=off
  Switch2 : Switch  Criteria=u2 ~= 0  OutMin=OutMin  OutMax=OutMax  OutDataTypeStr=Inherit: Inherit via back propagation  ZeroCross=off
  UpperRelop : RelationalOperator  DisableCoverage=on  Operator=<  OutDataTypeStr=boolean
  y : Outport  OutMin=OutMin  OutMax=OutMax
  wires:
  up/1 -> Switch2/1, LowerRelop1/2
  u/1 -> Data Type Propagation/2, Data Type Propagation/1, LowerRelop1/1, Switch/3, UpperRelop/1
  lo/1 -> Switch/1, UpperRelop/2
  Switch/1 -> Data Type Duplicate/2, Switch2/3, Data Type Propagation/3
  Switch2/1 -> Data Type Duplicate/1, y/1
  LowerRelop1/1 -> Switch2/2
  UpperRelop/1 -> Switch/2

== system Energy_converter_Electrical_to_Mechanical/e-Motor_chy_proposal/Umrichter mit trq-Regler/Umrechnung in el Leistung [W] ==
  note: Taken the output pwrTdcDes directly from here after multiplication . The switch output is now terminated
  trqEmot : Inport
  nEmot : Inport  Port=2
  dx/dt [m/s]1 : Gain  Gain=2*pi  SaturateOnIntegerOverflow=on  OutDataTypeStr=Inherit: Same as input  ParamDataTypeStr=Inherit: Same as input
      settings: AttributesFormatString=%<Gain>
  product1 : Product  SaturateOnIntegerOverflow=on  RndMeth=Zero  InputSameDT=on  OutDataTypeStr=Inherit: Same as first input
  pwrTdc : Outport
  wires:
  trqEmot/1 -> product1/1
  nEmot/1 -> dx/dt [m/s]1/1
  product1/1 -> pwrTdc/1  "pwrTdcDes"
  dx/dt [m/s]1/1 -> product1/2

== system Energy_converter_Electrical_to_Mechanical/e-Motor_chy_proposal/Umrichter mit trq-Regler/Umrechnung in el Leistung [W]_Max ==
  trqEmot : Inport
  nEmot : Inport  Port=2
  Abs : Abs
  Abs2 : Abs
  Eta Emot : Lookup_n-D  BreakpointsForDimension1=emot_pwrEtaTab_nRow  BreakpointsForDimension2=emot_pwrEtaTab_trqClm  Table=emot_pwrEtaTab_pwrTab  ExtrapMethod=Clip  SaturateOnIntegerOverflow=on  InputSameDT=on
  Gain1 : Gain  Gain=(emot_tractiongroup*2)
  Gain2 : Gain  Gain=1/(emot_tractiongroup*2)
  Gain4 : Gain  Gain=1/(emot_tractiongroup*2)
  Product1 : Product  Inputs=*/  SaturateOnIntegerOverflow=on  InputSameDT=on  OutDataTypeStr=Inherit: Same as first input
  const : Constant  Value=0
  dx/dt [m/s]1 : Gain  Gain=2*pi  SaturateOnIntegerOverflow=on  OutDataTypeStr=Inherit: Same as input  ParamDataTypeStr=Inherit: Same as input
      settings: AttributesFormatString=%<Gain>
  product : Product  SaturateOnIntegerOverflow=on  RndMeth=Zero  InputSameDT=on  OutDataTypeStr=Inherit: Same as first input
  product1 : Product  SaturateOnIntegerOverflow=on  RndMeth=Zero  InputSameDT=on  OutDataTypeStr=Inherit: Same as first input
  relational_operator : RelationalOperator  Operator=<=  InputSameDT=on
  switch : Switch  Threshold=0.5  SaturateOnIntegerOverflow=on  InputSameDT=on
      settings: AttributesFormatString=<threshold=%<threshold>>
  pwrTdc : Outport
  wires:
  Abs2/1 -> Eta Emot/1
  dx/dt [m/s]1/1 -> product1/2
  switch/1 -> Gain2/1  "pwrTdcDes"
  nEmot/1 -> dx/dt [m/s]1/1, Abs2/1
  Abs/1 -> Gain4/1
  Eta Emot/1 -> Product1/2, product/2  "eta"
  product1/1 -> Product1/1, product/1  "P"
  product/1 -> switch/1  "pwrRekup"
  Product1/1 -> switch/3  "pwrAntrieb"
  const/1 -> relational_operator/2
  relational_operator/1 -> switch/2
  trqEmot/1 -> Gain1/1
  Gain4/1 -> Eta Emot/2
  Gain1/1 -> product1/1, relational_operator/1, Abs/1
  Gain2/1 -> pwrTdc/1
